simulink model "Filtro_IIR_Butterworth_no_cuantizado"  (R2022a)
settings: Solver=ode4  StartTime=0.0  StopTime=Inf  FixedStep=1e-4  RelTol=1e-3  EnableMultiTasking=on
undefined symbols (not defined in the file): Gz
settings Model: ExtModeTrigDuration=8  Creator=05983057  LastModifiedBy=05983057
settings OptimizationCC: DefaultUnderspecifiedDataType=single  EnhancedBackFolding=on  PassReuseOutputArgsAs=Individual arguments  MaxStackSize=1024  OptimizeBlockOrder=speed  DifferentSizesBufferReuse=on  OptimizationCustomize=off  DenormalBehavior=FlushToZero  EfficientTunableParamExpr=on
settings DebuggingCC: ParameterTunabilityLossMsg=error
settings HardwareCC: ProdBitPerChar=16  ProdBitPerInt=16  ProdBitPerPointer=32  ProdBitPerSizeT=32  ProdBitPerPtrDiffT=32  ProdLargestAtomicInteger=Integer  ProdLargestAtomicFloat=None  ProdWordSize=16  ProdLongLongMode=on  ProdHWDeviceType=Texas Instruments->C2000
settings SFSimCC: MATLABDynamicMemAlloc=off
settings RTWCC: SystemTargetFile=ert.tlc  HardwareBoard=TI Delfino F2833x  TemplateMakefile=ert_default_tmf  Toolchain=Texas Instruments Code Composer Studio (C2000)
settings CodeAppCC: ForceParamTrailComments=on  IgnoreCustomStorageClasses=off  OperatorAnnotations=on  SimulinkDataObjDesc=on  SFDataObjDesc=on  InsertBlockDesc=on
settings ERTTargetCC: CodeReplacementLibrary=TI C28x  ExtModeTransport=3

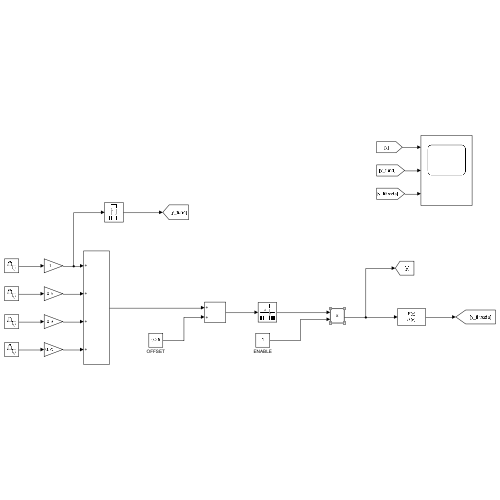
[thumbnail: Simulink's stored preview of the top-level diagram]
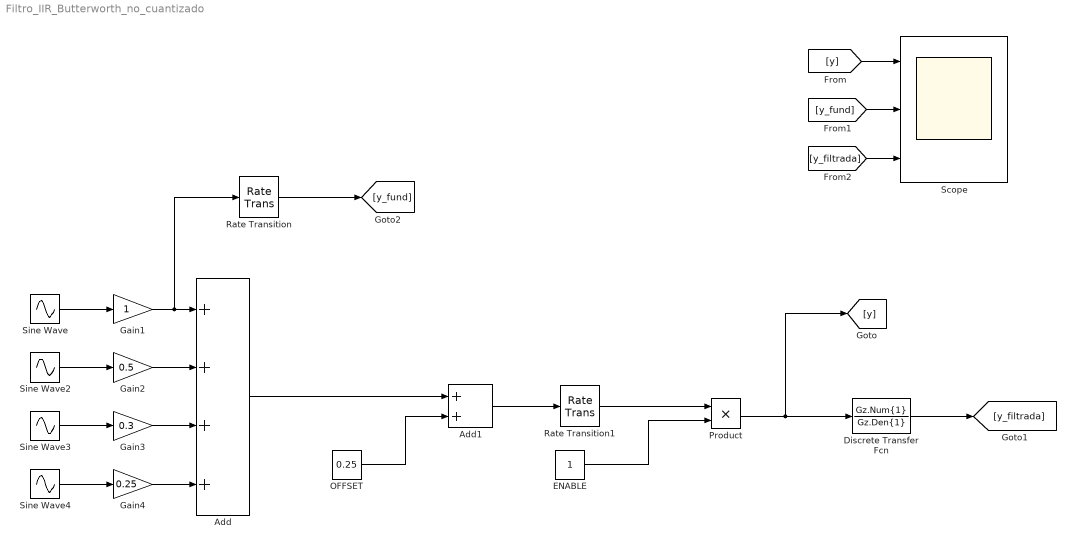
== system Filtro_IIR_Butterworth_no_cuantizado ==
  Add : Sum  Inputs=4
  Add1 : Sum  Inputs=2
  Discrete Transfer Fcn : DiscreteTransferFcn  Numerator=Gz.Num{1}  Denominator=Gz.Den{1}  SampleTime=1e-3
  ENABLE : Constant  SampleTime=1e-3
  Gain1 : Gain
  Gain2 : Gain  Gain=0.5
  Gain3 : Gain  Gain=0.3
  Gain4 : Gain  Gain=0.25
  OFFSET : Constant  Value=0.25  SampleTime=1e-4
  Product : Product
  Rate Transition : RateTransition  OutPortSampleTime=1e-3
  Rate Transition1 : RateTransition  OutPortSampleTime=1e-3
  Scope : Scope  NumInputPorts=3
  Sine Wave : Sin  Frequency=50*2*pi  SampleTime=1e-4
  Sine Wave2 : Sin  Frequency=150*2*pi  SampleTime=1e-4
  Sine Wave3 : Sin  Amplitude=0.3  Frequency=250*2*pi  SampleTime=1e-4
  Sine Wave4 : Sin  Frequency=350*2*pi  SampleTime=1e-4
  wires:
  Add/1 -> Add1/1
  Sine Wave/1 -> Gain1/1
  Rate Transition1/1 -> Product/1
  Add1/1 -> Rate Transition1/1
  Sine Wave4/1 -> Gain4/1
  Sine Wave3/1 -> Gain3/1
  OFFSET/1 -> Add1/2
  Sine Wave2/1 -> Gain2/1
  Gain3/1 -> Add/3
  Gain1/1 -> Rate Transition/1, Add/1
  [y] -> Scope/1
  Gain4/1 -> Add/4
  ENABLE/1 -> Product/2
  Gain2/1 -> Add/2
  Product/1 -> Discrete Transfer Fcn/1, [y]
  Rate Transition/1 -> [y_fund]
  [y_fund] -> Scope/2
  [y_filtrada] -> Scope/3
  Discrete Transfer Fcn/1 -> [y_filtrada]
